simulink model "TestCircle"  (R2018a)
settings: Solver=VariableStepAuto  StartTime=0.0  StopTime=10.0  RelTol=1e-3
libraries: simulink x2
settings Model: Creator=wangluo  LastModifiedBy=wangluo

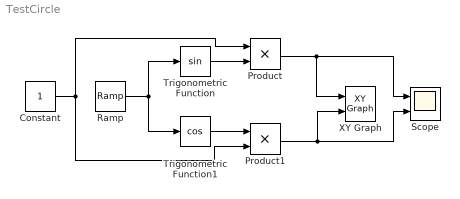
== system TestCircle ==
  Constant : Constant
  Product : Product
  Product1 : Product
  Ramp : simulink/Sources/Ramp  slope=1  start=0  InitialOutput=0
  Scope : Scope  NumInputPorts=2
  Trigonometric Function : Trigonometry
  Trigonometric Function1 : Trigonometry  Operator=cos
  XY Graph : simulink/Sinks/XY Graph  xmin=-1  xmax=1  ymin=-1  ymax=1  st=-1
  wires:
  Trigonometric Function/1 -> Product/2
  Trigonometric Function1/1 -> Product1/1
  Ramp/1 -> Trigonometric Function1/1, Trigonometric Function/1
  Constant/1 -> Product1/2, Product/1
  Product1/1 -> XY Graph/2, Scope/2
  Product/1 -> XY Graph/1, Scope/1
